simulink model "astr_hagg"  (R2020b)
settings: Solver=FixedStepAuto  StartTime=0.0  StopTime=300  FixedStep=0.1  RelTol=1e-3
undefined symbols (not defined in the file): k, r, T, tau
settings Model: Creator=Maciek  LastModifiedBy=Maciek

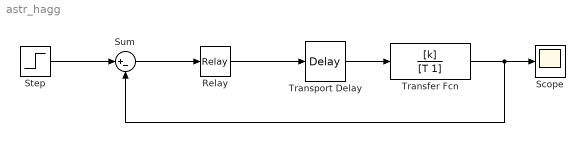
== system astr_hagg ==
  Relay : Relay  OnSwitchValue=0  OffSwitchValue=0  OnOutputValue=5  OffOutputValue=1
  Scope : Scope
  Step : Step  After=r  SampleTime=0
  Sum : Sum  Inputs=|+-
  Transfer Fcn : TransferFcn  Numerator=[k]  Denominator=[T 1]
  Transport Delay : TransportDelay  DelayTime=tau
  wires:
  Sum/1 -> Relay/1
  Step/1 -> Sum/1
  Transfer Fcn/1 -> Scope/1, Sum/2
  Relay/1 -> Transport Delay/1
  Transport Delay/1 -> Transfer Fcn/1
